simulink library "battery_model_lib"  (R2022b)
settings: Solver=VariableStepAuto  StartTime=0.0  StopTime=10.0  RelTol=1e-3
settings Model: Creator=dr_pa  LastModifiedBy=dr_pa

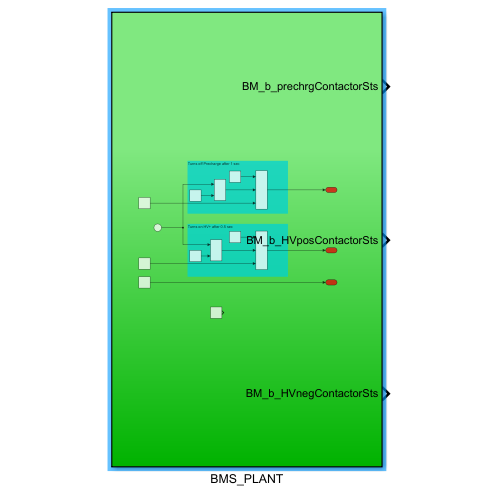
[thumbnail: Simulink's stored preview of the top-level diagram]
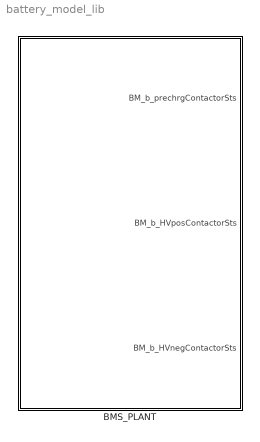
== system battery_model_lib ==
  BMS_PLANT : Subsystem

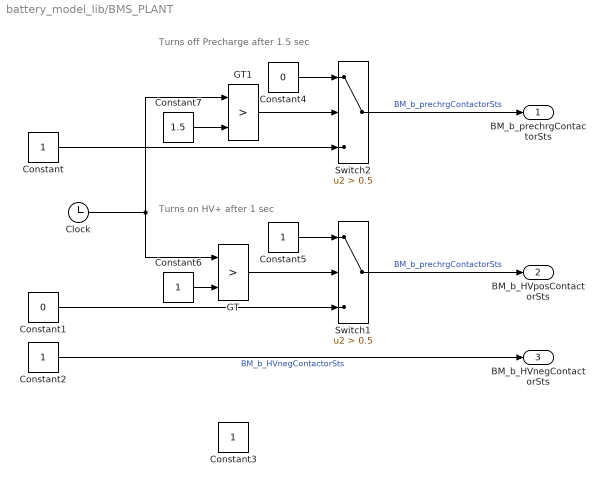
== system battery_model_lib/BMS_PLANT ==
  note: Turns off Precharge after 1.5 sec
  note: Turns on HV+ after 1 sec
  Clock : Clock
  Constant{,2..3,5..6} (5 alike) : Constant
  Constant1 : Constant  Value=0
  Constant4 : Constant  Value=0
  Constant7 : Constant  Value=1.5
  GT : RelationalOperator  Operator=>  OutDataTypeStr=boolean  RndMeth=Simplest  InputSameDT=off
  GT1 : RelationalOperator  Operator=>  OutDataTypeStr=boolean  RndMeth=Simplest  InputSameDT=off
  Switch1 : Switch  Criteria=u2 > Threshold  Threshold=0.5  SaturateOnIntegerOverflow=off  InputSameDT=off
  Switch2 : Switch  Criteria=u2 > Threshold  Threshold=0.5  SaturateOnIntegerOverflow=off  InputSameDT=off
  BM_b_prechrgContactorSts : Outport
  BM_b_HVposContactorSts : Outport  Port=2
  BM_b_HVnegContactorSts : Outport  Port=3
  wires:
  Switch2/1 -> BM_b_prechrgContactorSts/1  "BM_b_prechrgContactorSts"
  Constant2/1 -> BM_b_HVnegContactorSts/1  "BM_b_HVnegContactorSts"
  Constant4/1 -> Switch2/1
  Clock/1 -> GT1/1, GT/1
  Switch1/1 -> BM_b_HVposContactorSts/1  "BM_b_prechrgContactorSts"
  Constant1/1 -> Switch1/3
  Constant5/1 -> Switch1/1
  GT/1 -> Switch1/2
  Constant6/1 -> GT/2
  GT1/1 -> Switch2/2
  Constant7/1 -> GT1/2
  Constant/1 -> Switch2/3
